simulink model "first_test"  (R2023b)
settings: Solver=FixedStepAuto  StartTime=0.0  StopTime=10.0  RelTol=1e-3
PreLoadFcn:
  | % NXP_MBDT_S32K3 callback: DO NOT REMOVE
  | mbd_s32k3.common.nxp.model_callbacks.preLoadFcn();
PostLoadFcn:
  | % NXP_MBDT_S32K3 callback: DO NOT REMOVE
  | mbd_s32k3.common.nxp.model_callbacks.postLoadFcn();
InitFcn:
  | % NXP_MBDT_S32K3 callback: DO NOT REMOVE
  | mbd_s32k3.common.nxp.model_callbacks.initFcn();
libraries: mbd_s32k3_io_library x7
settings Model: DataDictionary=first_test.sldd  Creator=OWNER  LastModifiedBy=OWNER
settings OptimizationCC: EnhancedBackFolding=on  PassReuseOutputArgsAs=Individual arguments  ZeroExternalMemoryAtStartup=off  ZeroInternalMemoryAtStartup=off  MaxStackSize=64  OptimizeBlockOrder=speed  DifferentSizesBufferReuse=on  OptimizationCustomize=off  EfficientTunableParamExpr=on
settings DebuggingCC: InheritedTsInSrcMsg=none  ParameterTunabilityLossMsg=error
settings HardwareCC: ProdBitPerPointer=32  ProdBitPerSizeT=32  ProdBitPerPtrDiffT=32  ProdLargestAtomicInteger=Long  ProdLargestAtomicFloat=Double  ProdWordSize=32  ProdHWDeviceType=ARM Compatible->ARM Cortex
settings SFSimCC: MATLABDynamicMemAlloc=off
settings RTWCC: Description=Embedded Coder  SystemTargetFile=ert.tlc  HardwareBoard=NXP S32K3xx  TemplateMakefile=ert_default_tmf  GenerateReport=on  Toolchain=S32DS GCC
settings CodeAppCC: ForceParamTrailComments=on  IgnoreCustomStorageClasses=off  OperatorAnnotations=on  SimulinkDataObjDesc=on  SFDataObjDesc=on  InsertBlockDesc=on
settings ERTTargetCC: ExtModeTransport=1  ExtModeMexFile=ext_serial_win32_comm  ERTSrcFileBannerTemplate=mbd_s32k3_ert_code_template.cgt  ERTHdrFileBannerTemplate=mbd_s32k3_ert_code_template.cgt  ERTDataSrcFileTemplate=mbd_s32k3_ert_code_template.cgt  ERTDataHdrFileTemplate=mbd_s32k3_ert_code_template.cgt

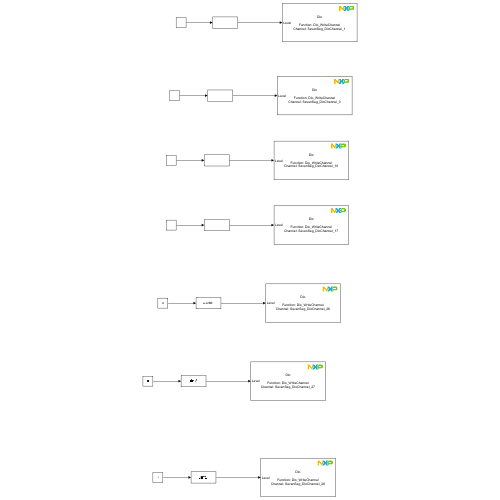
[thumbnail: Simulink's stored preview of the top-level diagram]
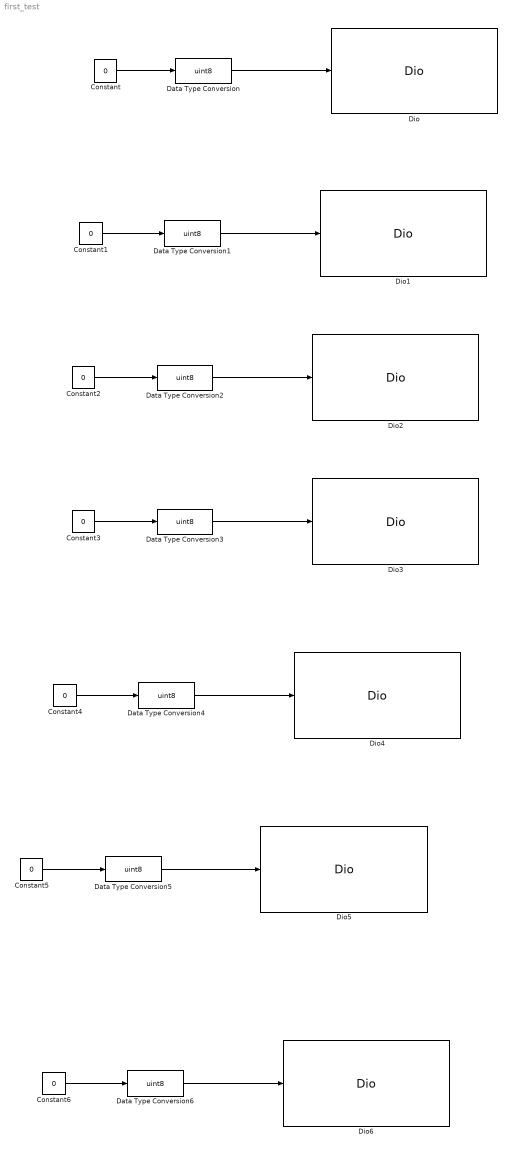
== system first_test ==
  Constant{,1..6} (7 alike) : Constant  Value=0
  Data Type Conversion{,1..6} (7 alike) : DataTypeConversion  OutDataTypeStr=uint8  SaturateOnIntegerOverflow=off  RndMeth=Floor
  Dio : mbd_s32k3_io_library/Dio  api_func=Dio_WriteChannel  channel=SevenSeg_DioChannel_1  channel_group=No channel groups configured  port=PTA_21  gpioSim=on  text=<binary blob, 2461 chars, not shown>
  Dio1 : mbd_s32k3_io_library/Dio  api_func=Dio_WriteChannel  channel=SevenSeg_DioChannel_0  channel_group=No channel groups configured  port=PTA_21  gpioSim=on  text=<binary blob, 2461 chars, not shown>
  Dio2 : mbd_s32k3_io_library/Dio  api_func=Dio_WriteChannel  channel=SevenSeg_DioChannel_10  channel_group=No channel groups configured  port=PTA_21  gpioSim=on  text=<binary blob, 2461 chars, not shown>
  Dio3 : mbd_s32k3_io_library/Dio  api_func=Dio_WriteChannel  channel=SevenSeg_DioChannel_17  channel_group=No channel groups configured  port=PTA_21  gpioSim=on  text=<binary blob, 2461 chars, not shown>
  Dio4 : mbd_s32k3_io_library/Dio  api_func=Dio_WriteChannel  channel=SevenSeg_DioChannel_26  channel_group=No channel groups configured  port=PTA_21  gpioSim=on  text=<binary blob, 2461 chars, not shown>
  Dio5 : mbd_s32k3_io_library/Dio  api_func=Dio_WriteChannel  channel=SevenSeg_DioChannel_27  channel_group=No channel groups configured  port=PTA_21  gpioSim=on  text=<binary blob, 2461 chars, not shown>
  Dio6 : mbd_s32k3_io_library/Dio  api_func=Dio_WriteChannel  channel=SevenSeg_DioChannel_28  channel_group=No channel groups configured  port=PTA_21  gpioSim=on  text=<binary blob, 2461 chars, not shown>
  wires:
  Constant/1 -> Data Type Conversion/1
  Data Type Conversion/1 -> Dio/1
  Constant1/1 -> Data Type Conversion1/1
  Data Type Conversion1/1 -> Dio1/1
  Constant2/1 -> Data Type Conversion2/1
  Data Type Conversion2/1 -> Dio2/1
  Constant3/1 -> Data Type Conversion3/1
  Data Type Conversion3/1 -> Dio3/1
  Constant4/1 -> Data Type Conversion4/1
  Data Type Conversion4/1 -> Dio4/1
  Constant5/1 -> Data Type Conversion5/1
  Data Type Conversion5/1 -> Dio5/1
  Constant6/1 -> Data Type Conversion6/1
  Data Type Conversion6/1 -> Dio6/1
